simulink model "Model_ref_ques7"  (R2020b)
settings: Solver=VariableStepAuto  StartTime=0.0  StopTime=10.0  RelTol=1e-3
settings Model: Creator=sneha  LastModifiedBy=sneha
settings DataIOCC: SaveOutput=off  SaveTime=off

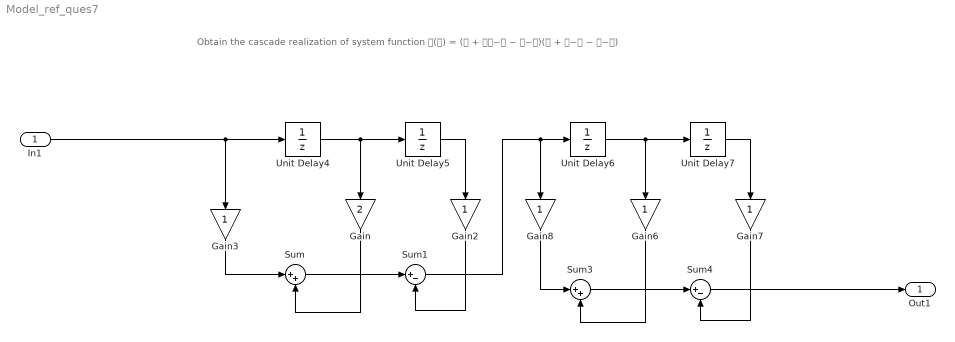
== system Model_ref_ques7 ==
  note: Obtain the cascade realization of system function 𝐇(𝐳) = (𝟏 + 𝟐𝐳−𝟏 − 𝐳−𝟐)(𝟏 + 𝐳−𝟏 − 𝐳−𝟐)
  In1 : Inport  OutDataTypeStr=double  PortDimensions=1  SampleTime=[0,1]
  Gain : Gain  Gain=2
  Gain{2..3,6..8} (5 alike) : Gain
  Sum : Sum  Inputs=|++
  Sum1 : Sum  Inputs=|+-
  Sum3 : Sum  Inputs=|++
  Sum4 : Sum  Inputs=|+-
  Unit Delay{4..7} (4 alike) : UnitDelay  SampleTime=-1  HasFrameUpgradeWarning=on
  Out1 : Outport  OutDataTypeStr=double  PortDimensions=1  SampleTime=[0,1]
  wires:
  Sum/1 -> Sum1/1
  Gain3/1 -> Sum/1
  Gain6/1 -> Sum3/2
  Unit Delay7/1 -> Gain7/1
  Unit Delay4/1 -> Unit Delay5/1, Gain/1
  Unit Delay5/1 -> Gain2/1
  Gain2/1 -> Sum1/2
  Gain8/1 -> Sum3/1
  Gain/1 -> Sum/2
  Gain7/1 -> Sum4/2
  In1/1 -> Gain3/1, Unit Delay4/1
  Sum1/1 -> Unit Delay6/1, Gain8/1
  Unit Delay6/1 -> Gain6/1, Unit Delay7/1
  Sum3/1 -> Sum4/1
  Sum4/1 -> Out1/1
